simulink model "Global_control_with_arbitraty_rate_of_convergence"  (R2021a)
settings: Solver=FixedStepDiscrete  StartTime=0.0  StopTime=12  FixedStep=1.0E-5  RelTol=1e-3
undefined symbols (not defined in the file): DiscIntNeverNeededParam, sigbuilder_block
libraries: simulink x4
(part 2 of 2)

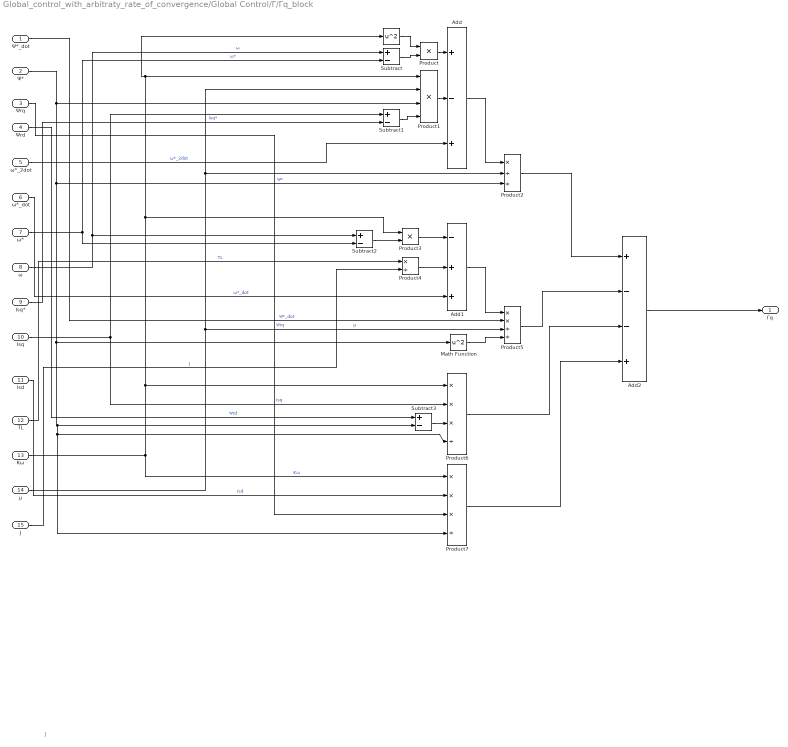
== system Global_control_with_arbitraty_rate_of_convergence/Global Control/Γ/Γq_block ==
  note: J
  Ψ*_dot : Inport
  Ψ* : Inport  Port=2
  Ψrq : Inport  Port=3
  Ψrd : Inport  Port=4
  ω*_2dot : Inport  Port=5
  ω*_dot : Inport  Port=6
  ω* : Inport  Port=7
  ω : Inport  Port=8
  Isq* : Inport  Port=9
  Isq : Inport  Port=10
  Isd : Inport  Port=11
  TL : Inport  Port=12
  Kω : Inport  Port=13
  µ : Inport  Port=14
  J : Inport  Port=15
  " " : Math  Operator=square  SaturateOnIntegerOverflow=on
  Add : Sum  Inputs=+-+
  Add1 : Sum  Inputs=-++
  Add2 : Sum  Inputs=+--+
  Math Function : Math  Operator=square  SaturateOnIntegerOverflow=on
  Product : Product
  Product1 : Product  Inputs=4
  Product2 : Product  Inputs=*//
  Product3 : Product
  Product4 : Product  Inputs=*/
  Product5 : Product  Inputs=**//
  Product6 : Product  Inputs=***/
  Product7 : Product  Inputs=***/
  Subtract{,1..3} (4 alike) : Sum  Inputs=+-
  Γq : Outport
  wires:
  Product7/1 -> Add2/4
  " "/1 -> Product/1
  Subtract2/1 -> Product3/2
  Ψ*/1 -> Product1/3, Product2/3, Subtract3/2, Product7/4, Product6/4, Math Function/1  "Ψ*"
  ω/1 -> Subtract2/1, Subtract/1  "ω"
  Ψrd/1 -> Subtract3/1  "Ψrd"
  Product1/1 -> Add/2
  Add1/1 -> Product5/1
  Product/1 -> Add/1
  µ/1 -> Product5/3, Product2/2, Product1/2  "µ"
  Subtract1/1 -> Product1/4
  ω*/1 -> Subtract2/2, Subtract/2  "ω*"
  Add2/1 -> Γq/1
  Kω/1 -> Product7/1, Product6/1, " "/1, Product1/1, Product3/1  "Kω"
  Product5/1 -> Add2/2
  Isq/1 -> Product6/2, Subtract1/1  "Isq"
  Product4/1 -> Add1/2
  Product6/1 -> Add2/3
  Subtract3/1 -> Product6/3
  Ψ*_dot/1 -> Product5/2  "Ψ*_dot"
  Isq*/1 -> Subtract1/2  "Isq*"
  Product2/1 -> Add2/1
  Ψrq/1 -> Product7/3  "Ψrq"
  Add/1 -> Product2/1
  Product3/1 -> Add1/1
  Subtract/1 -> Product/2
  Isd/1 -> Product7/2  "Isd"
  J/1 -> Product4/2  "J"
  Math Function/1 -> Product5/4
  TL/1 -> Product4/1  "TL"
  ω*_dot/1 -> Add1/3  "ω*_dot"
  ω*_2dot/1 -> Add/3  "ω*_2dot"
